simulink model "bai30"  (R2014a)
settings: Solver=ode45  StartTime=0.0  StopTime=10.0  RelTol=1e-3
settings Model: Creator=Lan  LastModifiedBy=Lan

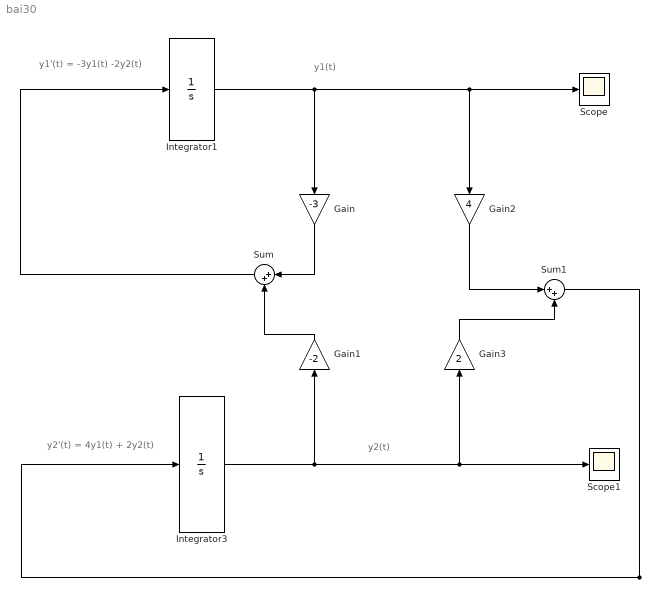
== system bai30 ==
  note: y2(t)
  note: y1(t)
  note: y2'(t) = 4y1(t) + 2y2(t)
  note: y1'(t) = -3y1(t) -2y2(t)
  Gain : Gain  Gain=-3
  Gain1 : Gain  Gain=-2
  Gain2 : Gain  Gain=4
  Gain3 : Gain  Gain=2
  Integrator1 : Integrator  InitialCondition=1
  Integrator3 : Integrator  InitialCondition=1
  Scope : Scope
  Scope1 : Scope
  Sum : Sum  Inputs=|++
  Sum1 : Sum  Inputs=|++
  wires:
  Integrator1/1 -> Gain/1, Gain2/1, Scope/1
  Integrator3/1 -> Gain1/1, Scope1/1, Gain3/1
  Gain1/1 -> Sum/2
  Gain/1 -> Sum/1
  Sum/1 -> Integrator1/1
  Gain2/1 -> Sum1/1
  Gain3/1 -> Sum1/2
  Sum1/1 -> Integrator3/1
